simulink model "Linearized_compensator"  (R2021b)
settings: Solver=VariableStepAuto  StartTime=0.0  StopTime=8  RelTol=1e-3
values from neighbouring files (symbols this model uses):
  eq = [0, 0, pi, 0]    [Linearization_comparison.m]    (also in Synthesis.m = [0, 0, -perturbation, 0]; init.m)
  K = acker(A, B, P)    [Synthesis.m]
  L_obs = temp'    [Synthesis.m]
  theta = pi    (= 3.14159265359)    [Synthesis.m]
undefined symbols (not defined in the file or in its folder): A, B, C, D
settings Model: Creator=brizio  LastModifiedBy=brizio

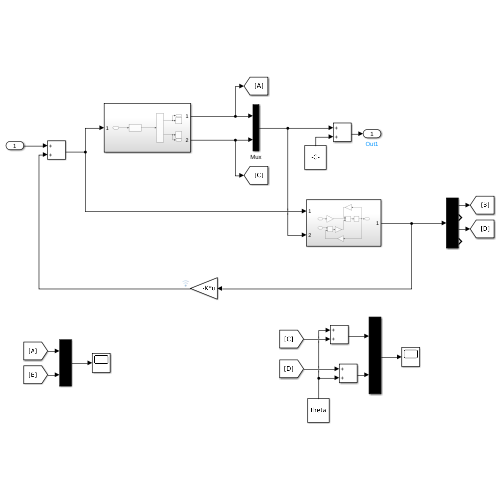
[thumbnail: Simulink's stored preview of the top-level diagram]
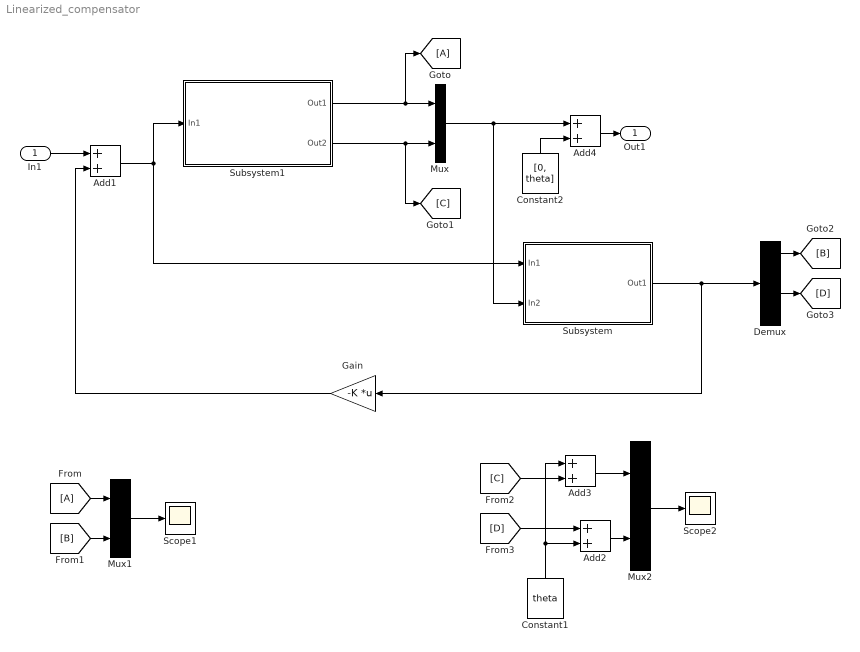
== system Linearized_compensator ==
  In1 : Inport
  Add{1..4} (4 alike) : Sum
  Constant1 : Constant  Value=theta
  Constant2 : Constant  Value=[0, theta]
  Demux : Demux
  Gain : Gain  Gain=-K  Multiplication=Matrix(K*u)
  Mux : Mux  Inputs=2
  Mux1 : Mux  Inputs=2
  Mux2 : Mux  Inputs=2
  Scope1 : Scope
  Scope2 : Scope
  Subsystem : Subsystem
  Subsystem1 : Subsystem
  Out1 : Outport
  wires:
  Subsystem/1(Out1) -> Demux/1, Gain/1
  Subsystem1/1(Out1) -> [A], Mux/1
  Mux/1 -> Add4/1, Subsystem/2(In2)
  Subsystem1/2(Out2) -> [C], Mux/2
  Mux1/1 -> Scope1/1
  [A] -> Mux1/1
  [B] -> Mux1/2
  Demux/1 -> [B]
  Demux/3 -> [D]
  Add2/1 -> Mux2/2
  Mux2/1 -> Scope2/1
  Add3/1 -> Mux2/1
  [D] -> Add2/1
  [C] -> Add3/2
  Constant1/1 -> Add2/2, Add3/1
  In1/1 -> Add1/1
  Gain/1 -> Add1/2
  Add1/1 -> Subsystem/1(In1), Subsystem1/1(In1)
  Constant2/1 -> Add4/2
  Add4/1 -> Out1/1

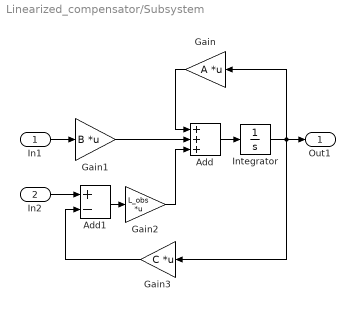
== system Linearized_compensator/Subsystem ==
  In1 : Inport
  In2 : Inport  Port=2
  Add : Sum  Inputs=+++
  Add1 : Sum  Inputs=+-
  Gain : Gain  Gain=A  Multiplication=Matrix(K*u)
  Gain1 : Gain  Gain=B  Multiplication=Matrix(K*u)
  Gain2 : Gain  Gain=L_obs  Multiplication=Matrix(K*u)
  Gain3 : Gain  Gain=C  Multiplication=Matrix(K*u)
  Integrator : Integrator
  Out1 : Outport
  wires:
  Add/1 -> Integrator/1
  In1/1 -> Gain1/1
  Gain/1 -> Add/1
  Gain1/1 -> Add/2
  Gain2/1 -> Add/3
  Add1/1 -> Gain2/1
  In2/1 -> Add1/1
  Gain3/1 -> Add1/2
  Integrator/1 -> Gain3/1, Gain/1, Out1/1

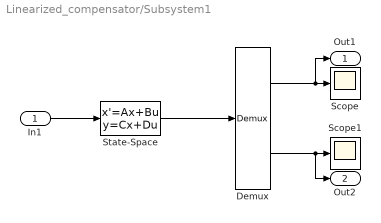
== system Linearized_compensator/Subsystem1 ==
  In1 : Inport
  Demux : Demux  Outputs=2
      settings: DisplayOption=none
  Scope : Scope
  Scope1 : Scope
  State-Space : StateSpace  A=A  B=B  C=C  D=D  InitialCondition=eq
  Out1 : Outport
  Out2 : Outport  Port=2
  wires:
  Demux/1 -> Out1/1, Scope/1
  Demux/2 -> Out2/1, Scope1/1
  State-Space/1 -> Demux/1
  In1/1 -> State-Space/1
